simulink model "motore_posizione_s"  (R2018b)
settings: Solver=VariableStepAuto  StartTime=0.0  StopTime=30.0  RelTol=1e-3
values from neighbouring files (symbols this model uses):
  A = [-11 -2.5 0;4 0 0;0 0.25 0]    [ex1.m]    (also in ex2.m; ex3.m = sys_s.a; ex4.m = sys_s.A; ex5.m = sys_c.A)
  B = [4 0 0]'    [ex1.m]    (also in ex2.m; ex3.m = sys_s.b; ex4.m = sys_s.B; ex5.m = sys_c.B)
  C = [0 0 5]    [ex1.m]    (also in ex2.m; ex3.m = sys_s.c; ex4.m = sys_s.C; ex5.m = sys_c.C)
  H = -acker(A',C',[lam_o lam_o lam_o*10])'    [ex7.m]    (also in ex8.m; motore.m = -acker(A',C',[lam_o lam_o])'; motore_posizione.m = -acker(A',C',[lam_o1 lam_o2 lam_o1])')
  J = 10    [motore_posizione.m]
  K = -acker(A,B,lam_d)    [ex1.m]    (also in ex2.m; ex3.m = -acker(A,B,lam_ds); ex4.m; ex5.m)
  k_d = 2    [ex2.m]    (also in ex3.m; ex4.m; ex5.m; ex6.m)
  k_i = Kt(4)    [ex4.m]    (also in ex5.m = T*Kt(4); ex6.m = T*Kt(4); motore_posizione.m)
  k_istar = T*Ktstar(4)    [motore_posizione.m]
  k_w = k_d/k_F    [ex2.m]    (also in ex3.m; ex4.m; ex5.m; ex6.m)
  k_wstar = k_d/k_Fstar    [ex3.m]    (also in ex8.m; motore_posizione.m = k_d/k_F)
  k_x = Kt(1:3)    [ex4.m]    (also in ex5.m; ex6.m; motore_posizione.m)
  k_xstar = Ktstar(1:3)    [motore_posizione.m]
  Kstar = -acker(Astar,Bstar,lam_dz)    [ex3.m]    (also in ex8.m; motore_posizione.m = -acker(Astar,Bstar,lam_dstar))
  T = 0.5/20    (= 0.025)    [ex3.m]    (also in ex5.m = 0.1; ex6.m = 0.2; ex8.m = 0.15; motore_posizione.m = 0.3)
settings Model: Creator=michelemaresca  LastModifiedBy=michelemaresca

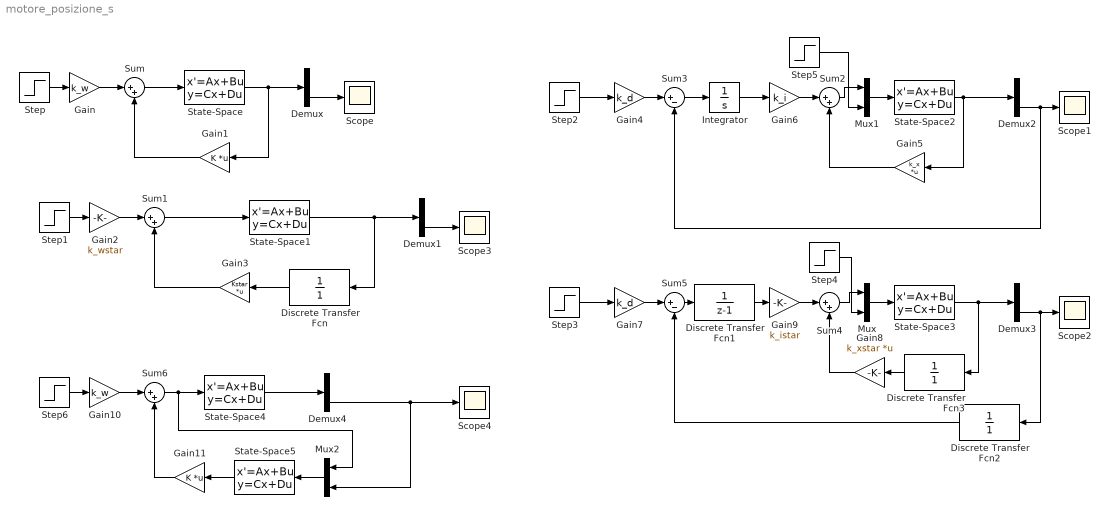
== system motore_posizione_s ==
  Demux{,1..4} (5 alike) : Demux  Outputs=3
  Discrete Transfer Fcn : DiscreteTransferFcn  Denominator=[1]  SampleTime=T
  Discrete Transfer Fcn1 : DiscreteTransferFcn  Denominator=[1 -1]  SampleTime=T
  Discrete Transfer Fcn2 : DiscreteTransferFcn  Denominator=[1]  SampleTime=T
  Discrete Transfer Fcn3 : DiscreteTransferFcn  Denominator=[1]  SampleTime=T
  Gain : Gain  Gain=k_w
  Gain1 : Gain  Gain=K  Multiplication=Matrix(K*u)
  Gain10 : Gain  Gain=k_w
  Gain11 : Gain  Gain=K  Multiplication=Matrix(K*u)
  Gain2 : Gain  Gain=k_wstar
  Gain3 : Gain  Gain=Kstar  Multiplication=Matrix(K*u)
  Gain4 : Gain  Gain=k_d
  Gain5 : Gain  Gain=k_x  Multiplication=Matrix(K*u)
  Gain6 : Gain  Gain=k_i
  Gain7 : Gain  Gain=k_d
  Gain8 : Gain  Gain=k_xstar  Multiplication=Matrix(K*u)
  Gain9 : Gain  Gain=k_istar
  Integrator : Integrator
  Mux : Mux  Inputs=2
  Mux1 : Mux  Inputs=2
  Mux2 : Mux  Inputs=2
  Scope{,1..4} (5 alike) : Scope
  State-Space : StateSpace  A=A  B=B  C=eye(3)  D=zeros(3,1)  InitialCondition=0
  State-Space1 : StateSpace  A=A  B=B  C=eye(3)  D=zeros(3,1)  InitialCondition=0
  State-Space2 : StateSpace  A=A  B=[B [0;-1/J;0]]  C=eye(3)  D=zeros(3,2)  InitialCondition=0
  State-Space3 : StateSpace  A=A  B=[B [0;-1/J;0]]  C=eye(3)  D=zeros(3,2)  InitialCondition=0
  State-Space4 : StateSpace  A=A  B=B  C=eye(3)  D=zeros(3,1)  InitialCondition=0
  State-Space5 : StateSpace  A=A+H*C  B=[B -H]  C=eye(3)  D=zeros(3,2)  InitialCondition=[0 0 pi/8]
  Step : Step  Time=0  SampleTime=0
  Step1 : Step  Time=0  SampleTime=T
  Step2 : Step  Time=0  SampleTime=0
  Step3 : Step  Time=0  SampleTime=T
  Step4 : Step  Time=10  After=40  SampleTime=T
  Step5 : Step  Time=10  After=40  SampleTime=0
  Step6 : Step  Time=0  SampleTime=0
  Sum{,1..2,4,6} (5 alike) : Sum  Inputs=|++
  Sum3 : Sum  Inputs=|+-
  Sum5 : Sum  Inputs=|+-
  wires:
  Step/1 -> Gain/1
  Gain/1 -> Sum/1
  Sum/1 -> State-Space/1
  State-Space/1 -> Gain1/1, Demux/1
  Gain1/1 -> Sum/2
  Gain3/1 -> Sum1/2
  Gain2/1 -> Sum1/1
  Step1/1 -> Gain2/1
  Sum1/1 -> State-Space1/1
  Discrete Transfer Fcn/1 -> Gain3/1
  Gain5/1 -> Sum2/2
  Step2/1 -> Gain4/1
  Gain4/1 -> Sum3/1
  Sum3/1 -> Integrator/1
  Gain6/1 -> Sum2/1
  Demux/3 -> Scope/1
  Demux1/3 -> Scope3/1
  State-Space1/1 -> Demux1/1, Discrete Transfer Fcn/1
  Demux2/3 -> Sum3/2, Scope1/1
  State-Space2/1 -> Gain5/1, Demux2/1
  Integrator/1 -> Gain6/1
  Discrete Transfer Fcn1/1 -> Gain9/1
  Step3/1 -> Gain7/1
  Gain7/1 -> Sum5/1
  Gain9/1 -> Sum4/1
  Demux3/3 -> Discrete Transfer Fcn2/1, Scope2/1
  Gain8/1 -> Sum4/2
  State-Space3/1 -> Discrete Transfer Fcn3/1, Demux3/1
  Sum5/1 -> Discrete Transfer Fcn1/1
  Discrete Transfer Fcn2/1 -> Sum5/2
  Sum4/1 -> Mux/1
  Mux/1 -> State-Space3/1
  Step4/1 -> Mux/2
  Sum2/1 -> Mux1/1
  Mux1/1 -> State-Space2/1
  Step5/1 -> Mux1/2
  Step6/1 -> Gain10/1
  Gain10/1 -> Sum6/1
  Sum6/1 -> Mux2/1, State-Space4/1
  State-Space4/1 -> Demux4/1
  Demux4/3 -> Mux2/2, Scope4/1
  Gain11/1 -> Sum6/2
  State-Space5/1 -> Gain11/1
  Mux2/1 -> State-Space5/1
  Discrete Transfer Fcn3/1 -> Gain8/1
